simulink model "crane_model"  (R2018b)
settings: Solver=VariableStepAuto  StartTime=0.0  StopTime=inf  FixedStep=0.001  RelTol=1e-3
values from neighbouring files (symbols this model uses):
  ba_c = Jeq_c * wv_c    [crane_constants.m]
  ba_i = Jeq_i * wv_i    [crane_constants.m]
  bcx = 1000    [crane_constants.m]
  bcy = 500    [crane_constants.m]
  beq_c = beq_c    (= 30)    [crane_constants.m]
  beq_i = beq_i    (= 18)    [crane_constants.m]
  Bw = 30    [crane_constants.m]
  g = 9.80665    [crane_constants.m]    (also in model_parameters.m)
  i_c = 15    [crane_constants.m]
  i_i = 30    [crane_constants.m]
  Jeq_c = (Mc*(Rw^2)/(i_c^2))+(Jw/(i_c^2))+Jm_c    (= 65.5644444444)    [crane_constants.m]
  Jeq_i = (-M_ln*Rd^2/(i_i^2))+(Jd/i_i^2)+Jm_i    (= -10.6161111111)    [crane_constants.m]
  Kcy = 1.3e8    (= 130000000)    [crane_constants.m]
  kisa_c = ksa_c * wi_c    [crane_constants.m]
  kisa_i = ksa_i * wi_i    [crane_constants.m]
  ksa_c = ba_c * wpos_c    [crane_constants.m]
  ksa_i = ba_i * wpos_i    [crane_constants.m]
  Kw = 1800    [crane_constants.m]
  lh_0 = 10    [crane_constants.m]
  M_l0 = M_h    (= 15000)    [crane_constants.m]    (also in model_parameters.m)
  M_lmin = M_h + M_cmin    (= 17000)    [crane_constants.m]    (also in model_parameters.m)
  M_ln = M_h + M_cn    (= 65000)    [crane_constants.m]    (also in model_parameters.m)
  Rd = 0.75    [crane_constants.m]
  Rw = 0.5    [crane_constants.m]
  Tau = 0.001    [crane_constants.m]    (also in cuatro_cuadr_const.m)
  xl_0 = 10    [crane_constants.m]
  xt_0 = 10    [crane_constants.m]
  y0 = 45    [crane_constants.m]
  yl_0 = 10    [crane_constants.m]
undefined symbols (not defined in the file or in its folder): ba_a, ksa_a, sXMax, sXMin, sYMax, sYMin
libraries: vrlib x1
settings Model: PauseTimes=3  Creator=Tincho  LastModifiedBy=Jere

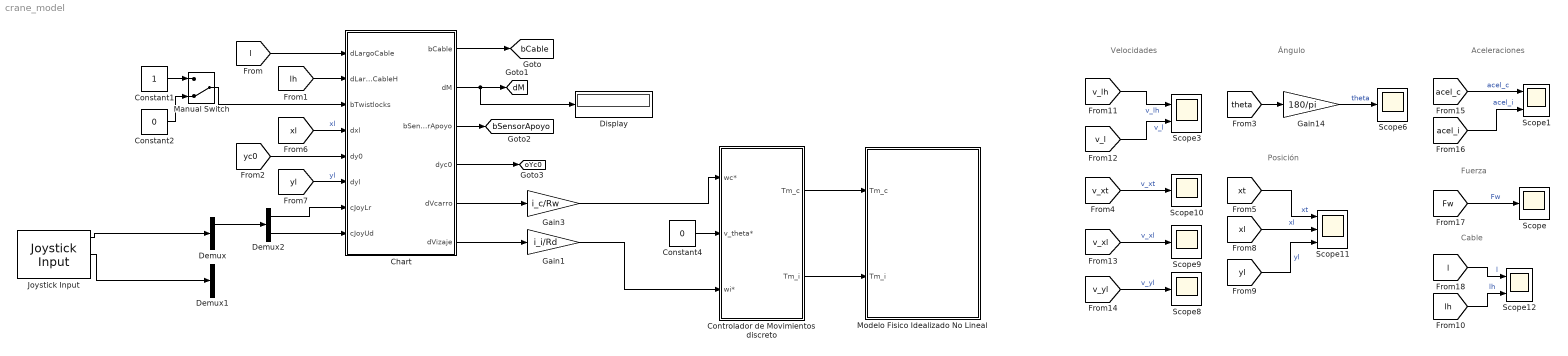
== system crane_model ==
  note: Cable
  note: Velocidades
  note: Fuerza
  note: Ángulo
  note: Posición
  note: Aceleraciones
  Chart : Stateflow chart  TreatAsAtomicUnit=on
  Constant1 : Constant  OutDataTypeStr=boolean
  Constant2 : Constant  Value=0  OutDataTypeStr=boolean
  Constant4 : Constant  Value=0
  Controlador de Movimientos discreto : Subsystem
  Demux : Demux  Outputs=2
  Demux1 : Demux  Outputs=2
  Demux2 : Demux  Outputs=2
  Display : Display
  Gain1 : Gain  Gain=i_i/Rd
  Gain14 : Gain  Gain=180/pi
  Gain3 : Gain  Gain=i_c/Rw
  Joystick Input : vrlib/Joystick Input  joyid=1  adjustports=on  forcefeed=off
      settings: SourceProductBaseCode=VR
  Manual Switch : ManualSwitch  CurrentSetting=0
  Modelo Fisico Idealizado No Lineal : Subsystem
  Scope{,6,8..10} (5 alike) : Scope
  Scope1 : Scope  NumInputPorts=2
  Scope11 : Scope  NumInputPorts=3
  Scope12 : Scope  NumInputPorts=2
  Scope3 : Scope  NumInputPorts=2
  tag scope: bCable=global, bSensorApoyo=global, dM=global, oYc0=global
  wires:
  [l] -> Chart/1(dLargoCable)
  [lh] -> Chart/2(dLargoCableH)
  Manual Switch/1 -> Chart/3(bTwistlocks)
  Constant1/1 -> Manual Switch/1
  Constant2/1 -> Manual Switch/2
  Chart/2(dM) -> Display/1, [dM]
  [yc0] -> Chart/5(dy0)
  Chart/3(bSensorApoyo) -> [bSensorApoyo]
  [xl] -> Chart/4(dxl)  "xl"
  [yl] -> Chart/6(dyl)  "yl"
  Chart/4(dyc0) -> [oYc0]
  Chart/1(bCable) -> [bCable]
  Joystick Input/1 -> Demux/1
  Joystick Input/2 -> Demux1/1
  Chart/6(dVizaje) -> Gain1/1
  Chart/5(dVcarro) -> Gain3/1
  Demux/1 -> Demux2/1
  Demux2/2 -> Chart/8(cJoyUd)
  Demux2/1 -> Chart/7(cJoyLr)
  [v_xt] -> Scope10/1  "v_xt"
  [lh] -> Scope12/2  "lh"
  [v_lh] -> Scope3/1  "v_lh"
  [xl] -> Scope11/2  "xl"
  [v_l] -> Scope3/2  "v_l"
  [acel_i] -> Scope1/2  "acel_i"
  [xt] -> Scope11/1  "xt"
  [acel_c] -> Scope1/1  "acel_c"
  [Fw] -> Scope/1  "Fw"
  [l] -> Scope12/1  "l"
  [theta] -> Gain14/1
  Gain3/1 -> Controlador de Movimientos discreto/1(wc*)
  Gain14/1 -> Scope6/1  "theta"
  Controlador de Movimientos discreto/1(Tm_c) -> Modelo Fisico Idealizado No Lineal/1(Tm_c)
  [v_xl] -> Scope9/1  "v_xl"
  [v_yl] -> Scope8/1  "v_yl"
  [yl] -> Scope11/3  "yl"
  Controlador de Movimientos discreto/2(Tm_i) -> Modelo Fisico Idealizado No Lineal/2(Tm_i)
  Constant4/1 -> Controlador de Movimientos discreto/2(v_theta*)
  Gain1/1 -> Controlador de Movimientos discreto/3(wi*)

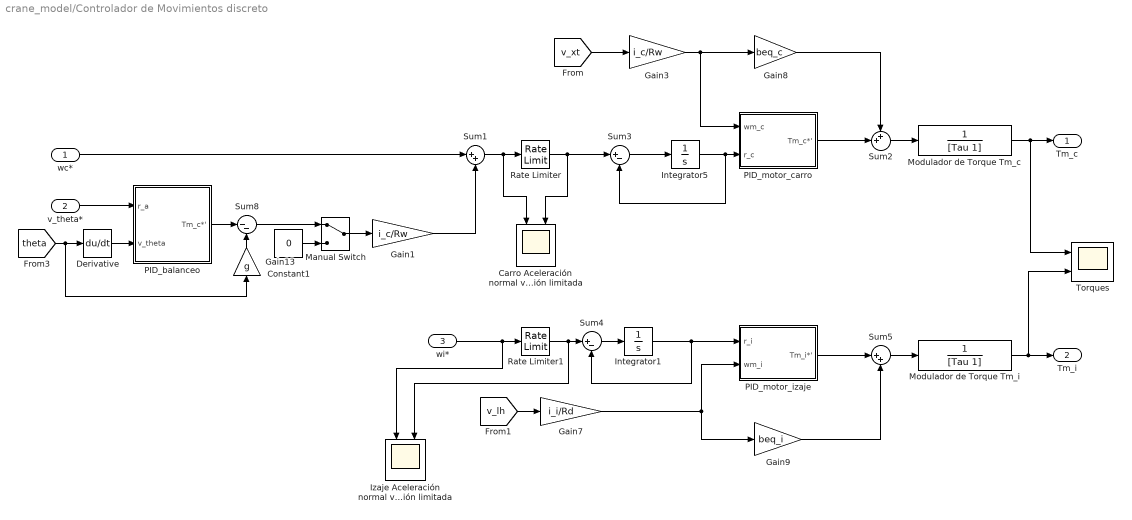
== system crane_model/Controlador de Movimientos discreto ==
  wc* : Inport
  v_theta* : Inport  Port=2
  wi* : Inport  Port=3
  "             Izaje Aceleración normal vs Aceleración limitada" : Scope  NumInputPorts=2
  "            Carro Aceleración normal vs Aceleración limitada" : Scope  NumInputPorts=2
  Constant1 : Constant  Value=0
  Derivative : Derivative  CoefficientInTFapproximation=0
  Gain1 : Gain  Gain=i_c/Rw
  Gain13 : Gain  Gain=g
  Gain3 : Gain  Gain=i_c/Rw
  Gain7 : Gain  Gain=i_i/Rd
  Gain8 : Gain  Gain=beq_c
  Gain9 : Gain  Gain=beq_i
  Integrator1 : Integrator
  Integrator5 : Integrator
  Manual Switch : ManualSwitch
  Modulador de Torque Tm_c : TransferFcn  Denominator=[Tau 1]
  Modulador de Torque Tm_i : TransferFcn  Denominator=[Tau 1]
  PID_balanceo : Subsystem
  PID_motor_carro : Subsystem
  PID_motor_izaje : Subsystem
  Rate Limiter : RateLimiter  RisingSlewLimit=1*i_c/Rw  FallingSlewLimit=-1*i_c/Rw  LinearizeAsGain=off
  Rate Limiter1 : RateLimiter  RisingSlewLimit=1*i_i/Rd  FallingSlewLimit=-1*i_i/Rd  LinearizeAsGain=off
  Sum1 : Sum  Inputs=|++
  Sum2 : Sum  Inputs=++|
  Sum3 : Sum  Inputs=|+-
  Sum4 : Sum  Inputs=|+-
  Sum5 : Sum  Inputs=|++
  Sum8 : Sum  Inputs=|--
  Torques : Scope  NumInputPorts=2
  Tm_c : Outport
  Tm_i : Outport  Port=2
  wires:
  wc*/1 -> Sum1/1
  Modulador de Torque Tm_i/1 -> Torques/2, Tm_i/1
  Sum5/1 -> Modulador de Torque Tm_i/1
  wi*/1 -> Rate Limiter1/1, "             Izaje Aceleración normal vs Aceleración limitada"/1
  Sum3/1 -> Integrator5/1
  Sum4/1 -> Integrator1/1
  Integrator5/1 -> Sum3/2, PID_motor_carro/2(r_c)
  Constant1/1 -> Manual Switch/2
  [theta] -> Gain13/1, Derivative/1
  Gain8/1 -> Sum2/1
  Rate Limiter1/1 -> "             Izaje Aceleración normal vs Aceleración limitada"/2, Sum4/1
  [v_lh] -> Gain7/1
  Gain13/1 -> Sum8/2
  Gain3/1 -> PID_motor_carro/1(wm_c), Gain8/1
  Sum8/1 -> Manual Switch/1
  Rate Limiter/1 -> "            Carro Aceleración normal vs Aceleración limitada"/2, Sum3/1
  Gain9/1 -> Sum5/2
  [v_xt] -> Gain3/1
  Manual Switch/1 -> Gain1/1
  Derivative/1 -> PID_balanceo/2(v_theta)
  Gain7/1 -> PID_motor_izaje/2(wm_i), Gain9/1
  Sum1/1 -> "            Carro Aceleración normal vs Aceleración limitada"/1, Rate Limiter/1
  Gain1/1 -> Sum1/2
  PID_motor_carro/1(Tm_c*') -> Sum2/2
  PID_motor_izaje/1(Tm_i*') -> Sum5/1
  PID_balanceo/1(Tm_c*') -> Sum8/1
  v_theta*/1 -> PID_balanceo/1(r_a)
  Sum2/1 -> Modulador de Torque Tm_c/1
  Modulador de Torque Tm_c/1 -> Tm_c/1, Torques/1
  Integrator1/1 -> Sum4/2, PID_motor_izaje/1(r_i)

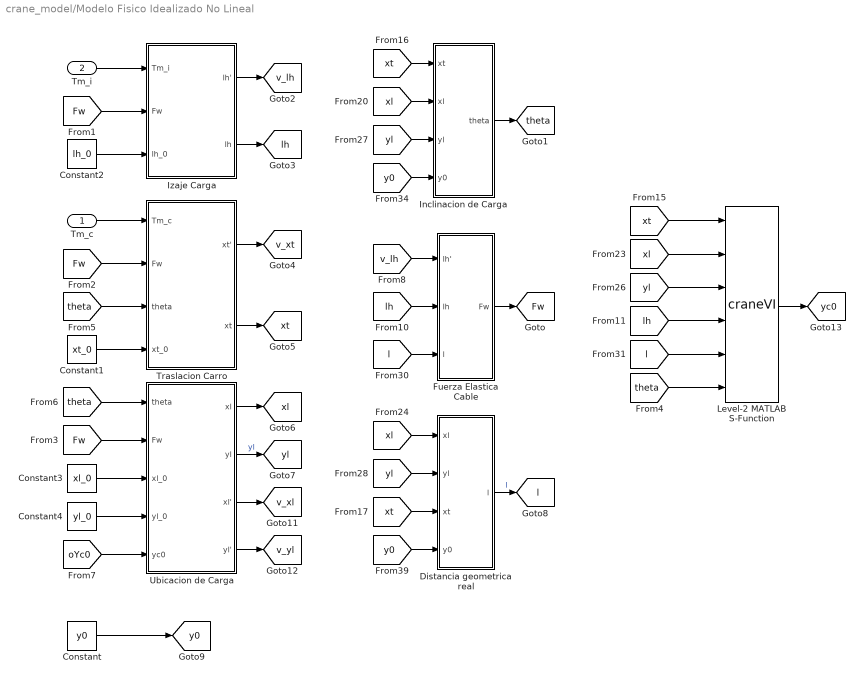
== system crane_model/Modelo Fisico Idealizado No Lineal ==
  Tm_c : Inport
  Tm_i : Inport  Port=2
  Constant : Constant  Value=y0
  Constant1 : Constant  Value=xt_0
  Constant2 : Constant  Value=lh_0
  Constant3 : Constant  Value=xl_0
  Constant4 : Constant  Value=yl_0
  Distancia geometrica real : Subsystem
  Fuerza Elastica Cable : Subsystem
  Inclinacion de Carga : Subsystem
  Izaje Carga : Subsystem
  Level-2 MATLAB S-Function : M-S-Function  FunctionName=craneVI  Parameters=xl_0, yl_0
  Traslacion Carro : Subsystem
  Ubicacion de Carga : Subsystem
  tag scope: Fw=global, l=global, lh=global, theta=global, v_lh=global, v_xl=global, v_xt=global, v_yl=global, xl=global, xt=global, y0=global, yc0=global, yl=global
  wires:
  Constant/1 -> [y0]
  Traslacion Carro/2(xt) -> [xt]
  Ubicacion de Carga/1(xl) -> [xl]
  Ubicacion de Carga/2(yl) -> [yl]  "yl"
  Distancia geometrica real/1(l) -> [l]  "l"
  Traslacion Carro/1(xt') -> [v_xt]
  Izaje Carga/2(lh) -> [lh]
  Izaje Carga/1(lh') -> [v_lh]
  Inclinacion de Carga/1(theta) -> [theta]
  Constant4/1 -> Ubicacion de Carga/4(yl_0)
  Constant3/1 -> Ubicacion de Carga/3(xl_0)
  Constant1/1 -> Traslacion Carro/4(xt_0)
  Constant2/1 -> Izaje Carga/3(lh_0)
  Tm_c/1 -> Traslacion Carro/1(Tm_c)
  Tm_i/1 -> Izaje Carga/1(Tm_i)
  Fuerza Elastica Cable/1(Fw) -> [Fw]
  [Fw] -> Izaje Carga/2(Fw)
  [Fw] -> Traslacion Carro/2(Fw)
  [Fw] -> Ubicacion de Carga/2(Fw)
  [theta] -> Level-2 MATLAB S-Function/6
  [theta] -> Traslacion Carro/3(theta)
  [theta] -> Ubicacion de Carga/1(theta)
  [v_lh] -> Fuerza Elastica Cable/1(lh')
  [lh] -> Fuerza Elastica Cable/2(lh)
  [lh] -> Level-2 MATLAB S-Function/4
  [xt] -> Level-2 MATLAB S-Function/1
  [xt] -> Inclinacion de Carga/1(xt)
  [xt] -> Distancia geometrica real/3(xt)
  [xl] -> Inclinacion de Carga/2(xl)
  [xl] -> Level-2 MATLAB S-Function/2
  [xl] -> Distancia geometrica real/1(xl)
  [yl] -> Level-2 MATLAB S-Function/3
  [yl] -> Inclinacion de Carga/3(yl)
  [yl] -> Distancia geometrica real/2(yl)
  [l] -> Fuerza Elastica Cable/3(l)
  [l] -> Level-2 MATLAB S-Function/5
  [y0] -> Inclinacion de Carga/4(y0)
  Ubicacion de Carga/3(xl') -> [v_xl]
  Ubicacion de Carga/4(yl') -> [v_yl]
  [y0] -> Distancia geometrica real/4(y0)
  Level-2 MATLAB S-Function/1 -> [yc0]
  [oYc0] -> Ubicacion de Carga/5(yc0)

== system crane_model/Controlador de Movimientos discreto/PID_balanceo ==
  r_a : Inport
  v_theta : Inport  Port=2
  Gain10 : Gain  Gain=ba_a
  Gain11 : Gain  Gain=ksa_a
  Integrator : Integrator
  Sum6 : Sum  Inputs=|+-
  Sum7 : Sum  Inputs=|++
  Tm_c*' : Outport
  wires:
  Sum6/1 -> Integrator/1, Gain10/1
  r_a/1 -> Sum6/1
  Integrator/1 -> Gain11/1
  Sum7/1 -> Tm_c*'/1
  v_theta/1 -> Sum6/2
  Gain11/1 -> Sum7/1
  Gain10/1 -> Sum7/2

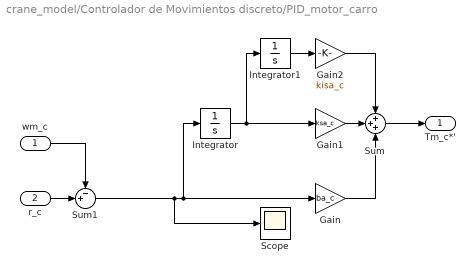
== system crane_model/Controlador de Movimientos discreto/PID_motor_carro ==
  wm_c : Inport
  r_c : Inport  Port=2
  Gain : Gain  Gain=ba_c
  Gain1 : Gain  Gain=ksa_c
  Gain2 : Gain  Gain=kisa_c
  Integrator : Integrator
  Integrator1 : Integrator
  Scope : Scope
  Sum : Sum  Inputs=+++
  Sum1 : Sum  Inputs=-+|
  Tm_c*' : Outport
  wires:
  Gain1/1 -> Sum/2
  Integrator/1 -> Gain1/1, Integrator1/1
  r_c/1 -> Sum1/2
  Gain2/1 -> Sum/1
  Integrator1/1 -> Gain2/1
  Gain/1 -> Sum/3
  wm_c/1 -> Sum1/1
  Sum/1 -> Tm_c*'/1
  Sum1/1 -> Gain/1, Integrator/1, Scope/1

== system crane_model/Controlador de Movimientos discreto/PID_motor_izaje ==
  r_i : Inport
  wm_i : Inport  Port=2
  Gain4 : Gain  Gain=ba_i
  Gain5 : Gain  Gain=ksa_i
  Gain6 : Gain  Gain=kisa_i
  Integrator2 : Integrator
  Integrator3 : Integrator
  Sum3 : Sum  Inputs=+++
  Sum4 : Sum  Inputs=|+-
  Tm_i*' : Outport
  wires:
  r_i/1 -> Sum4/1
  Integrator3/1 -> Gain6/1
  Sum4/1 -> Gain4/1, Integrator2/1
  Integrator2/1 -> Gain5/1, Integrator3/1
  wm_i/1 -> Sum4/2
  Gain5/1 -> Sum3/2
  Sum3/1 -> Tm_i*'/1
  Gain6/1 -> Sum3/3
  Gain4/1 -> Sum3/1

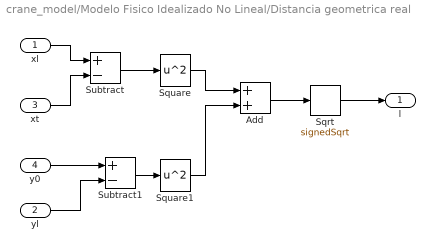
== system crane_model/Modelo Fisico Idealizado No Lineal/Distancia geometrica real ==
  xl : Inport
  yl : Inport  Port=2
  xt : Inport  Port=3
  y0 : Inport  Port=4
  Add : Sum
  Sqrt : Sqrt  Operator=signedSqrt  SaturateOnIntegerOverflow=on
  Square : Math  Operator=square  SaturateOnIntegerOverflow=on
  Square1 : Math  Operator=square  SaturateOnIntegerOverflow=on
  Subtract : Sum  Inputs=+-
  Subtract1 : Sum  Inputs=+-
  l : Outport
  wires:
  yl/1 -> Subtract1/2
  Square/1 -> Add/1
  y0/1 -> Subtract1/1
  Square1/1 -> Add/2
  Subtract1/1 -> Square1/1
  xt/1 -> Subtract/2
  Add/1 -> Sqrt/1
  Subtract/1 -> Square/1
  xl/1 -> Subtract/1
  Sqrt/1 -> l/1

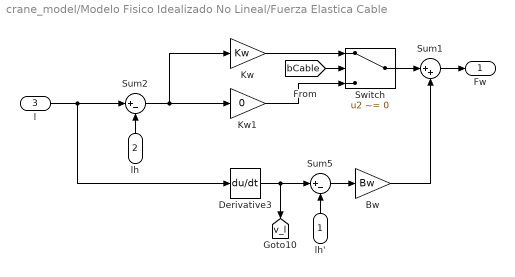
== system crane_model/Modelo Fisico Idealizado No Lineal/Fuerza Elastica Cable ==
  lh' : Inport
  lh : Inport  Port=2
  l : Inport  Port=3
  Bw : Gain  Gain=Bw
  Derivative3 : Derivative
  Kw : Gain  Gain=Kw
  Kw1 : Gain  Gain=0
  Sum1 : Sum  Inputs=|++
  Sum2 : Sum  Inputs=|+-
  Sum5 : Sum  Inputs=|+-
  Switch : Switch  Criteria=u2 ~= 0
  Fw : Outport
  tag scope: v_l=global
  wires:
  Sum5/1 -> Bw/1
  Bw/1 -> Sum1/2
  Kw/1 -> Switch/1
  lh'/1 -> Sum5/2
  l/1 -> Derivative3/1, Sum2/1
  Kw1/1 -> Switch/3
  lh/1 -> Sum2/2
  Switch/1 -> Sum1/1
  Sum2/1 -> Kw/1, Kw1/1
  Sum1/1 -> Fw/1
  Derivative3/1 -> Sum5/1, [v_l]
  [bCable] -> Switch/2

== system crane_model/Modelo Fisico Idealizado No Lineal/Inclinacion de Carga ==
  xt : Inport
  xl : Inport  Port=2
  yl : Inport  Port=3
  y0 : Inport  Port=4
  Atan2 : Trigonometry  Operator=atan2
  Subtract : Sum  Inputs=+-
  Subtract1 : Sum  Inputs=+-
  theta : Outport
  wires:
  xl/1 -> Subtract/1
  Subtract/1 -> Atan2/1
  y0/1 -> Subtract1/1
  Subtract1/1 -> Atan2/2
  xt/1 -> Subtract/2
  yl/1 -> Subtract1/2
  Atan2/1 -> theta/1

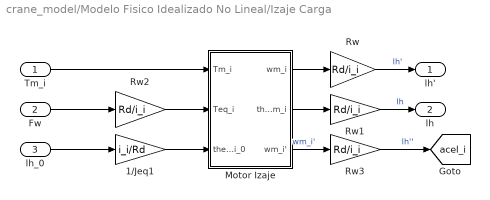
== system crane_model/Modelo Fisico Idealizado No Lineal/Izaje Carga ==
  Tm_i : Inport
  Fw : Inport  Port=2
  lh_0 : Inport  Port=3
  1/Jeq1 : Gain  Gain=i_i/Rd
  Motor Izaje : Subsystem
  Rw{,1..3} (4 alike) : Gain  Gain=Rd/i_i
  lh' : Outport
  lh : Outport  Port=2
  tag scope: acel_i=global
  wires:
  Motor Izaje/2(thetam_i) -> Rw1/1
  Rw2/1 -> Motor Izaje/2(Teq_i)
  Motor Izaje/1(wm_i) -> Rw/1
  Rw/1 -> lh'/1  "lh'"
  Rw1/1 -> lh/1  "lh"
  Tm_i/1 -> Motor Izaje/1(Tm_i)
  lh_0/1 -> 1/Jeq1/1
  Fw/1 -> Rw2/1
  1/Jeq1/1 -> Motor Izaje/3(theta_i_0)
  Rw3/1 -> [acel_i]  "lh''"
  Motor Izaje/3(wm_i') -> Rw3/1  "wm_i'"

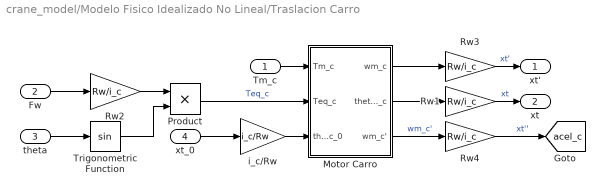
== system crane_model/Modelo Fisico Idealizado No Lineal/Traslacion Carro ==
  Tm_c : Inport
  Fw : Inport  Port=2
  theta : Inport  Port=3
  xt_0 : Inport  Port=4
  Motor Carro : Subsystem
  Product : Product
  Rw{1..4} (4 alike) : Gain  Gain=Rw/i_c
  Trigonometric Function : Trigonometry
  i_c/Rw : Gain  Gain=i_c/Rw
  xt' : Outport
  xt : Outport  Port=2
  tag scope: acel_c=global
  wires:
  theta/1 -> Trigonometric Function/1
  Motor Carro/2(thetam_c) -> Rw1/1
  Product/1 -> Motor Carro/2(Teq_c)  "Teq_c"
  Rw1/1 -> xt/1  "xt"
  Rw2/1 -> Product/1
  Tm_c/1 -> Motor Carro/1(Tm_c)
  Trigonometric Function/1 -> Product/2
  Fw/1 -> Rw2/1
  xt_0/1 -> i_c/Rw/1
  Motor Carro/1(wm_c) -> Rw3/1
  Rw3/1 -> xt'/1  "xt'"
  i_c/Rw/1 -> Motor Carro/3(theta_c_0)
  Rw4/1 -> [acel_c]  "xt''"
  Motor Carro/3(wm_c') -> Rw4/1  "wm_c'"

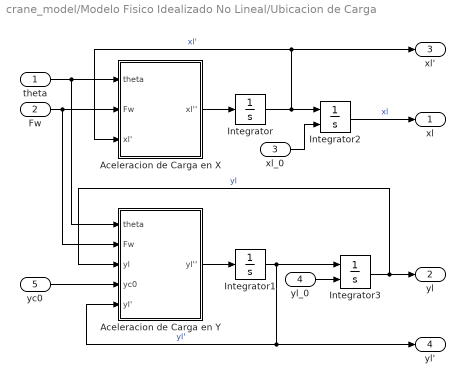
== system crane_model/Modelo Fisico Idealizado No Lineal/Ubicacion de Carga ==
  theta : Inport
  Fw : Inport  Port=2
  xl_0 : Inport  Port=3
  yl_0 : Inport  Port=4
  yc0 : Inport  Port=5
  Aceleracion de Carga en X : Subsystem
  Aceleracion de Carga en Y : Subsystem
  Integrator : Integrator
  Integrator1 : Integrator
  Integrator2 : Integrator  InitialConditionSource=external
  Integrator3 : Integrator  InitialConditionSource=external
  xl : Outport
  yl : Outport  Port=2
  xl' : Outport  Port=3
  yl' : Outport  Port=4
  wires:
  Aceleracion de Carga en Y/1(yl'') -> Integrator1/1
  Integrator3/1 -> Aceleracion de Carga en Y/3(yl), yl/1  "yl"
  Integrator/1 -> Aceleracion de Carga en X/3(xl'), xl'/1, Integrator2/1  "xl'"
  Fw/1 -> Aceleracion de Carga en X/2(Fw), Aceleracion de Carga en Y/2(Fw)
  Integrator2/1 -> xl/1  "xl"
  Integrator1/1 -> Aceleracion de Carga en Y/5(yl'), yl'/1, Integrator3/1  "yl'"
  Aceleracion de Carga en X/1(xl'') -> Integrator/1
  xl_0/1 -> Integrator2/2
  yl_0/1 -> Integrator3/2
  yc0/1 -> Aceleracion de Carga en Y/4(yc0)
  theta/1 -> Aceleracion de Carga en X/1(theta), Aceleracion de Carga en Y/1(theta)

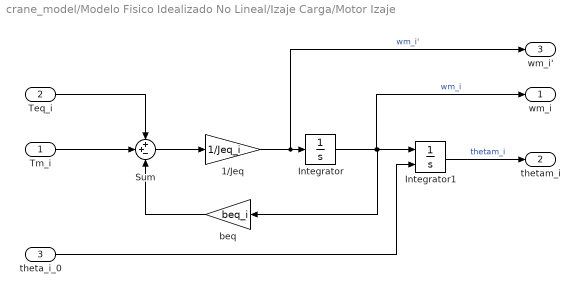
== system crane_model/Modelo Fisico Idealizado No Lineal/Izaje Carga/Motor Izaje ==
  Tm_i : Inport
  Teq_i : Inport  Port=2
  theta_i_0 : Inport  Port=3
  1/Jeq : Gain  Gain=1/Jeq_i
  Integrator : Integrator
  Integrator1 : Integrator  InitialConditionSource=external
  Sum : Sum  Inputs=++-
  beq : Gain  Gain=beq_i
  wm_i : Outport
  thetam_i : Outport  Port=2
  wm_i' : Outport  Port=3
  wires:
  Sum/1 -> 1/Jeq/1
  Integrator/1 -> wm_i/1, beq/1, Integrator1/1  "wm_i"
  Integrator1/1 -> thetam_i/1  "thetam_i"
  1/Jeq/1 -> wm_i'/1, Integrator/1  "wm_i'"
  beq/1 -> Sum/3
  theta_i_0/1 -> Integrator1/2
  Tm_i/1 -> Sum/2
  Teq_i/1 -> Sum/1

== system crane_model/Modelo Fisico Idealizado No Lineal/Traslacion Carro/Motor Carro ==
  Tm_c : Inport
  Teq_c : Inport  Port=2
  theta_c_0 : Inport  Port=3
  1/Jeq : Gain  Gain=1/Jeq_c
  Integrator : Integrator
  Integrator1 : Integrator  InitialConditionSource=external
  Sum : Sum  Inputs=++-
  beq : Gain  Gain=beq_c
  wm_c : Outport
  thetam_c : Outport  Port=2
  wm_c' : Outport  Port=3
  wires:
  Sum/1 -> 1/Jeq/1
  Integrator/1 -> wm_c/1, beq/1, Integrator1/1  "wm_c"
  Integrator1/1 -> thetam_c/1  "thetam_c"
  1/Jeq/1 -> wm_c'/1, Integrator/1  "wm_c'"
  beq/1 -> Sum/3
  theta_c_0/1 -> Integrator1/2
  Tm_c/1 -> Sum/2
  Teq_c/1 -> Sum/1

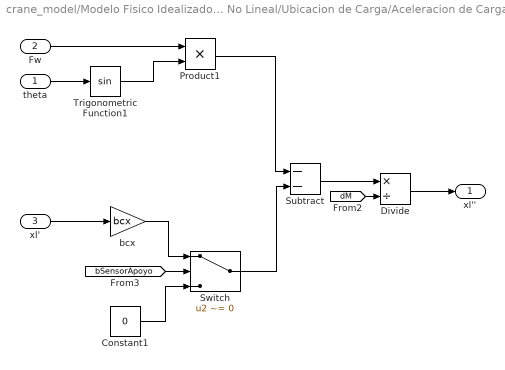
== system crane_model/Modelo Fisico Idealizado No Lineal/Ubicacion de Carga/Aceleracion de Carga en X ==
  theta : Inport
  Fw : Inport  Port=2
  xl' : Inport  Port=3
  Constant1 : Constant  Value=0
  Divide : Product  Inputs=*/
  Product1 : Product
  Subtract : Sum  Inputs=--
  Switch : Switch  Criteria=u2 ~= 0
  Trigonometric Function1 : Trigonometry
  bcx : Gain  Gain=bcx
  xl'' : Outport
  wires:
  Divide/1 -> xl''/1
  theta/1 -> Trigonometric Function1/1
  Switch/1 -> Subtract/2
  Fw/1 -> Product1/1
  Trigonometric Function1/1 -> Product1/2
  Product1/1 -> Subtract/1
  xl'/1 -> bcx/1
  Subtract/1 -> Divide/1
  bcx/1 -> Switch/1
  Constant1/1 -> Switch/3
  [dM] -> Divide/2
  [bSensorApoyo] -> Switch/2

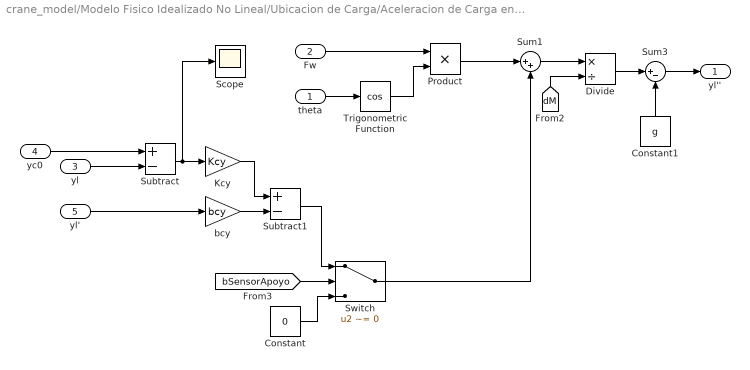
== system crane_model/Modelo Fisico Idealizado No Lineal/Ubicacion de Carga/Aceleracion de Carga en Y ==
  theta : Inport
  Fw : Inport  Port=2
  yl : Inport  Port=3
  yc0 : Inport  Port=4
  yl' : Inport  Port=5
  Constant : Constant  Value=0
  Constant1 : Constant  Value=g
  Divide : Product  Inputs=*/
  Kcy : Gain  Gain=Kcy
  Product : Product
  Scope : Scope
  Subtract : Sum  Inputs=+-
  Subtract1 : Sum  Inputs=+-
  Sum1 : Sum  Inputs=|++
  Sum3 : Sum  Inputs=|+-
  Switch : Switch  Criteria=u2 ~= 0
  Trigonometric Function : Trigonometry  Operator=cos
  bcy : Gain  Gain=bcy
  yl'' : Outport
  wires:
  Fw/1 -> Product/1
  Trigonometric Function/1 -> Product/2
  Divide/1 -> Sum3/1
  Constant1/1 -> Sum3/2
  yl/1 -> Subtract/2
  Constant/1 -> Switch/3
  theta/1 -> Trigonometric Function/1
  Subtract1/1 -> Switch/1
  Subtract/1 -> Scope/1, Kcy/1
  yl'/1 -> bcy/1
  Kcy/1 -> Subtract1/1
  Product/1 -> Sum1/1
  Switch/1 -> Sum1/2
  Sum3/1 -> yl''/1
  bcy/1 -> Subtract1/2
  Sum1/1 -> Divide/1
  [dM] -> Divide/2
  [bSensorApoyo] -> Switch/2
  yc0/1 -> Subtract/1

== stateflow chart crane_model/Chart ==
  settings: executeAtInitialization=1
  state ComandosManuales [parallel]
    settings: executionOrder=5
    state MoveHoist [parallel]
      settings: executionOrder=2
      state MoveUpward
        du:
        dVizaje = -1;
      state Waiting
        en:
        dVizaje = 0;
      state Contact
        du:
        dVizaje = 0;
      state MoveDownward
        du:
        dVizaje = 1;
      ComandosManuales.MoveHoist.Waiting -> MoveUpward [order 1] : [cJoyUd == -1]
      Contact -> MoveUpward : [cJoyUd==-1]
      MoveUpward -> ComandosManuales.MoveHoist.Waiting : [cJoyUd == 0]
      (default) -> ComandosManuales.MoveHoist.Waiting
      MoveDownward -> ComandosManuales.MoveHoist.Waiting [order 1] : [cJoyUd == 0]
      ComandosManuales.MoveHoist.Waiting -> MoveDownward [order 2] : [cJoyUd == 1]
      MoveDownward -> Contact [order 2] : [bSensorApoyo]
    state MoveTrolly [parallel]
      settings: executionOrder=1
      state MoveForward
        du:
        dVcarro = 1;
      state Waiting
        du:
        dVcarro = 0;
      state MoveBackward
        du:
        dVcarro = -1;
      ComandosManuales.MoveTrolly.Waiting -> MoveForward [order 1] : [cJoyLr == 1]
      MoveForward -> ComandosManuales.MoveTrolly.Waiting : [cJoyLr == 0]
      (default) -> ComandosManuales.MoveTrolly.Waiting
      ComandosManuales.MoveTrolly.Waiting -> MoveBackward [order 2] : [cJoyLr == -1]
      MoveBackward -> ComandosManuales.MoveTrolly.Waiting : [cJoyLr == 0]
  state Cable [parallel]
    settings: executionOrder=1
    state NoApoyado
      entry:
      bCable=true;
    state Apoyado
      entry:
      bCable=false;
    (default) -> NoApoyado
    NoApoyado -> Apoyado : [ 0 < (dLargoCableH - dLargoCable)]
    Apoyado -> NoApoyado : [ 0 >= (dLargoCableH - dLargoCable)]
  state SensorApoyo [parallel]
    settings: executionOrder=4
    state Activado
      en:
      bAux=false;
      bSensorApoyo = true;
      dyc0 = dPerfilObstaculos(dxl,dy0);
      on after(1,sec): bAux= true;
    state Desactivado
      en:
      bSensorApoyo = false;
      during:
      dyc0 = dPerfilObstaculos(dxl,dy0);
    (default) -> Desactivado
    Desactivado -> Activado : [ 0 <= dyc0 - dyl ]
    Activado -> Desactivado : [ 0 > dyc0 - dyl && bAux]
  state LimitesDeMovimientosCarro [parallel]
    settings: executionOrder=6
    state FinDeCarreraOff
      entry:
      bFCarCarro = false;
    state FinDeCarrera_Stop
      entry:
      bFCarCarro = true;
    (default) -> LimitesDeMovimientosCarro.FinDeCarreraOff
    LimitesDeMovimientosCarro.FinDeCarreraOff -> LimitesDeMovimientosCarro.FinDeCarrera_Stop : [sXMax<=dxl || dxl<=sXMin]
  state LimitesDeMovimientosIzaje [parallel]
    settings: executionOrder=7
    state FinDeCarreraOff
      entry:
      bFCarIzaje = false;
    state FinDeCarrera_Stop
      entry:
      bFCarIzaje = true;
    (default) -> LimitesDeMovimientosIzaje.FinDeCarreraOff
    LimitesDeMovimientosIzaje.FinDeCarreraOff -> LimitesDeMovimientosIzaje.FinDeCarrera_Stop : [sYMax<=dyl || dyl<=sYMin]
  note: Este bloque representa la funcionalidad de toma y liberecion de carga.
      | Tal vez, más adelante haya que implementar un estado entre medio para
      | habilitar al operario a cerrar los twitslocks y elevar el gancho vacio en el
      | orden correspondiente. (Estilo automata de seguridad).
      | Otra posibilidad es implementarlo en el estado donde se setea el bSensorApoyo.
      | Apoyo -> Trabo Destrabo -> Retiro
  state Spreader [parallel]
    settings: executionOrder=2
    state Vacio
      en:
      bSprCargado = false;
      dM = M_l0;
    state Cargado
      en:
      bSprCargado = true;
      dM = M_ln ;
    (default) -> Spreader.Vacio
    Spreader.Cargado -> Spreader.Vacio : [~bTwistlocks && ~bSensorApoyo]
    Spreader.Vacio -> Spreader.Cargado : [bTwistlocks && bSensorApoyo]
  state VelocidadesMaximas [parallel]
    settings: executionOrder=3
    state Vacio
      en:
      dVmax_i = 3.0;
    state Cargado
      en:
      dVmax_i = -1.5 * dM / M_ln + 3;
      dVmax_i = round(dVmax_i * 1000) / 1000;
    (default) -> VelocidadesMaximas.Vacio
    VelocidadesMaximas.Vacio -> VelocidadesMaximas.Cargado : [bSprCargado]
    VelocidadesMaximas.Cargado -> VelocidadesMaximas.Vacio : [~bSprCargado]
  data: xl_ function_input; y0_ function_input; yc0_ function_output; bSprCargado local boolean =false; dLargoCable input double; dLargoCableH input double; bCable output boolean; bTwistlocks input boolean; M_ln parameter double; M_lmin parameter double; dM output double; M_l0 parameter double; dxl input double; dy0 input; dyl input double; bSensorApoyo output boolean; dyc0 output double =0; dVcarro output double; dVizaje output double; cJoyLr input double; cJoyUd input double; dVmax_i local double; bAux local; sXMax parameter double; sXMin parameter double; sYMax parameter double; sYMin parameter double
  function yc0_ = dPerfilObstaculos(xl_, y0_):
    | function yc0_ = dPerfilObstaculos(xl_, y0_)
    | w = 5;   %width
    | nMaxContX = 9; %cantidad maxima de columnas de containers
    | dx = 2;
    | yc0_ = 0;
    | if xl_ <= -2
    |     yc0_ = 0;
    | elseif xl_ > -2 && xl_ <= 2
    |     yc0_ = 15;
    | elseif xl_ > 48
    |     yc0_ = 0;
    | else
    |     for i = 1:nMaxContX
    |         if xl_ > dx && xl_ <= dx+w
    | %             
    |             yc0_ = y0_(i);
    | %            
    |             break;
    |         end
    |         dx = dx+w;
    |     end
    | end
    | % disp('yc0');
    | % disp(yc0_);
    | end
